simulink model "switch_control_Led"  (R2022b)
settings: Solver=FixedStepDiscrete  StartTime=0.0  StopTime=20  FixedStep=0.001  RelTol=1e-3
libraries: pil_lib x1
settings Model: Creator=Dell  LastModifiedBy=Dell
settings DataIOCC: OutputSaveName=MIL_output  LoggingToFile=on  LoggingFileName=MIL_output.mat
settings OptimizationCC: DefaultParameterBehavior=Inlined  UseDivisionForNetSlopeComputation=on  GainParamInheritBuiltInType=on  UseFloatMulNetSlope=on  InlineInvariantSignals=on  PassReuseOutputArgsAs=Individual arguments  ZeroExternalMemoryAtStartup=off  ZeroInternalMemoryAtStartup=off  NoFixptDivByZeroProtection=on  EfficientFloat2IntCast=on  LifeSpan=1  OptimizeBlockOrder=speed  DifferentSizesBufferReuse=on  EfficientTunableParamExpr=on
settings DebuggingCC: ParameterTunabilityLossMsg=error
settings HardwareCC: ProdBitPerPointer=32  ProdBitPerSizeT=32  ProdBitPerPtrDiffT=32  ProdLargestAtomicInteger=Long  ProdLargestAtomicFloat=Double  ProdWordSize=32  ProdLongLongMode=on  ProdHWDeviceType=ARM Compatible->ARM Cortex-M
settings SFSimCC: MATLABDynamicMemAlloc=off
settings RTWCC: Description=Embedded Coder  SystemTargetFile=ert.tlc  TemplateMakefile=ert_default_tmf
settings CodeAppCC: ForceParamTrailComments=on  IgnoreCustomStorageClasses=off  OperatorAnnotations=on  SimulinkDataObjDesc=on  SFDataObjDesc=on  CustomSymbolStrGlobalVar=rt$N$M  CustomSymbolStrType=$N$M  CustomSymbolStrFcn=$N$M$F  CustomSymbolStrMacro=$N$M  InsertBlockDesc=on
settings ERTTargetCC: TargetLangStandard=C99 (ISO)  GenerateSampleERTMain=on  IncludeMdlTerminateFcn=off  CombineSignalStateStructs=on  SuppressErrorStatus=on  SupportAbsoluteTime=off  SupportComplex=off  InlinedParameterPlacement=NonHierarchical  ERTCustomFileTemplate=example_file_process.tlc  ERTFilePackagingFormat=CompactWithDataFile

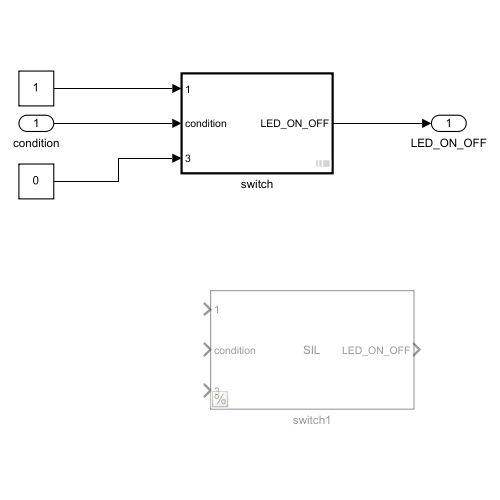
[thumbnail: Simulink's stored preview of the top-level diagram]
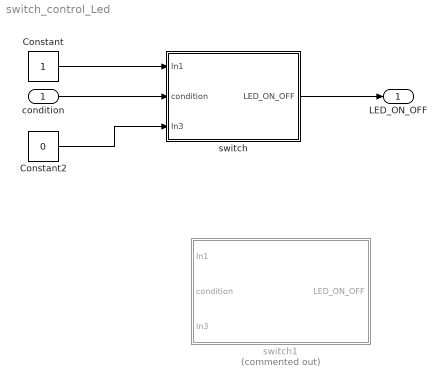
== system switch_control_Led ==
  condition : Inport
  Constant : Constant
  Constant2 : Constant  Value=0
  switch : Subsystem  TreatAsAtomicUnit=on
  switch1 : Subsystem  Tag=__SL_testing_harness_stub_  Commented=on  DialogController=pil_create_dialog  LoadFcn=|
      | try
      |    if ~strcmp(rtw.pil.getPILVersion, '9.13 (R2022b)_15')
      |       set_param(gcb, 'DialogController', '');
      |       set_param(gcb, 'DialogControllerArgs', '');
      |    end
      | catch e
      |       set_param(gcb, 'DialogController', '');
      |       set_param(gcb, 'DialogControllerArgs', '');
      | end
      mask help: PIL:pil:XILBlockMaskDesc
      mask Display: disp('SIL');
  LED_ON_OFF : Outport
  wires:
  condition/1 -> switch/2(condition)
  Constant2/1 -> switch/3(In3)
  Constant/1 -> switch/1(In1)
  switch/1(LED_ON_OFF) -> LED_ON_OFF/1

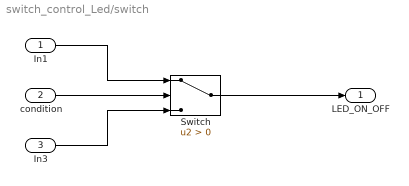
== system switch_control_Led/switch ==
  In1 : Inport
  condition : Inport  Port=2
  In3 : Inport  Port=3
  Switch : Switch  Criteria=u2 > Threshold  SaturateOnIntegerOverflow=off  InputSameDT=off
  LED_ON_OFF : Outport
  wires:
  condition/1 -> Switch/2
  Switch/1 -> LED_ON_OFF/1
  In3/1 -> Switch/3
  In1/1 -> Switch/1

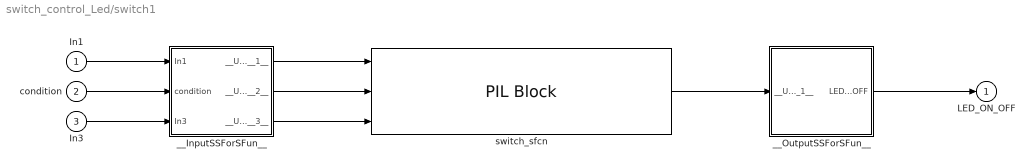
== system switch_control_Led/switch1 ==
  In1 : Inport
  condition : Inport  Port=2
  In3 : Inport  Port=3
  __InputSSForSFun__ : Subsystem
  __OutputSSForSFun__ : Subsystem
  switch_sfcn : pil_lib/PIL Block  SimulationMode=SIL  IsTopModelPIL=off  CodeDir=switch0_ert_rtw  AnchorDir=E:\MBD\Embedded_coder\switch_ON_OFF  ConfigName=Software-in-the-Loop (SIL)  XrelIsTopModelCode=on  XrelIsReusable=off  XrelDWorkNames={}  XrelDWorkTypes={}  XrelModelArgVals={}  XrelOrderedParamNames={}
  LED_ON_OFF : Outport
  wires:
  __OutputSSForSFun__/1(LED_ON_OFF) -> LED_ON_OFF/1
  switch_sfcn/1 -> __OutputSSForSFun__/1(__UniqueInportName__1__)
  __InputSSForSFun__/3(__UniqueOutportName__3__) -> switch_sfcn/3
  __InputSSForSFun__/2(__UniqueOutportName__2__) -> switch_sfcn/2
  __InputSSForSFun__/1(__UniqueOutportName__1__) -> switch_sfcn/1
  In3/1 -> __InputSSForSFun__/3(In3)
  condition/1 -> __InputSSForSFun__/2(condition)
  In1/1 -> __InputSSForSFun__/1(In1)

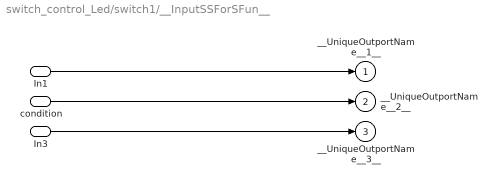
== system switch_control_Led/switch1/__InputSSForSFun__ ==
  In1 : Inport
  condition : Inport  Port=2
  In3 : Inport  Port=3
  __UniqueOutportName__1__ : Outport
  __UniqueOutportName__2__ : Outport  Port=2
  __UniqueOutportName__3__ : Outport  Port=3
  wires:
  In3/1 -> __UniqueOutportName__3__/1
  condition/1 -> __UniqueOutportName__2__/1
  In1/1 -> __UniqueOutportName__1__/1

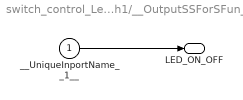
== system switch_control_Led/switch1/__OutputSSForSFun__ ==
  __UniqueInportName__1__ : Inport
  LED_ON_OFF : Outport
  wires:
  __UniqueInportName__1__/1 -> LED_ON_OFF/1
